simulink model "punto5a"  (R2018b)
settings: Solver=VariableStepAuto  StartTime=0.0  StopTime=10.0  RelTol=1e-3
libraries: neural x3
settings Model: Creator=seba  LastModifiedBy=seba

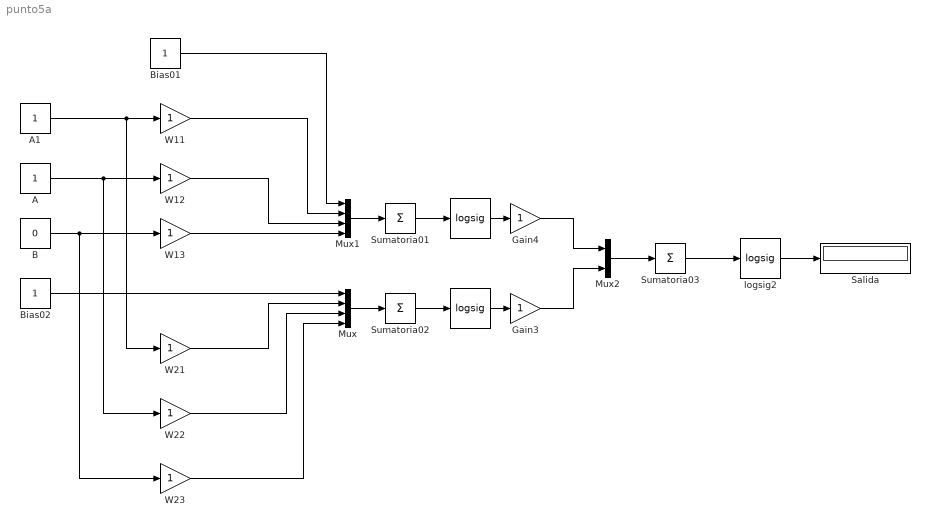
== system punto5a ==
  " " : neural/Transfer Functions/logsig
      settings: SourceProductName=Neural Network Toolbox  SourceProductBaseCode=NN
  " " : neural/Transfer Functions/logsig
      settings: SourceProductName=Neural Network Toolbox  SourceProductBaseCode=NN
  A : Constant
  A1 : Constant
  "B " : Constant  Value=0
  "Bias01 " : Constant
  "Bias02 " : Constant
  Gain3 : Gain
  Gain4 : Gain
  Mux : Mux
  Mux1 : Mux
  Mux2 : Mux  Inputs=2
  "Salida " : Display
  "Sumatoria01 " : Sum  Inputs=+
  "Sumatoria02 " : Sum  Inputs=+
  "Sumatoria03 " : Sum  Inputs=+
  "W11 " : Gain
  "W12 " : Gain
  "W13 " : Gain
  "W21 " : Gain
  W22 : Gain
  "W23 " : Gain
  logsig2 : neural/Transfer Functions/logsig
      settings: SourceProductName=Neural Network Toolbox  SourceProductBaseCode=NN
  wires:
  "W21 "/1 -> Mux/2
  W22/1 -> Mux/3
  "W23 "/1 -> Mux/4
  "Bias02 "/1 -> Mux/1
  Mux/1 -> "Sumatoria02 "/1
  "Sumatoria02 "/1 -> " "/1
  " "/1 -> Gain3/1
  " "/1 -> Gain4/1
  "Sumatoria01 "/1 -> " "/1
  Mux1/1 -> "Sumatoria01 "/1
  "W13 "/1 -> Mux1/4
  "W12 "/1 -> Mux1/3
  "W11 "/1 -> Mux1/2
  "Bias01 "/1 -> Mux1/1
  A1/1 -> "W21 "/1, "W11 "/1
  A/1 -> "W12 "/1, W22/1
  "B "/1 -> "W23 "/1, "W13 "/1
  Gain4/1 -> Mux2/1
  Gain3/1 -> Mux2/2
  Mux2/1 -> "Sumatoria03 "/1
  "Sumatoria03 "/1 -> logsig2/1
  logsig2/1 -> "Salida "/1
